simulink model "DisplayCANMsg"  (R2015a)
settings: Solver=ode45  StartTime=0.0  StopTime=10000000.0  RelTol=1e-3
settings Model: Creator=t430  LastModifiedBy=t430

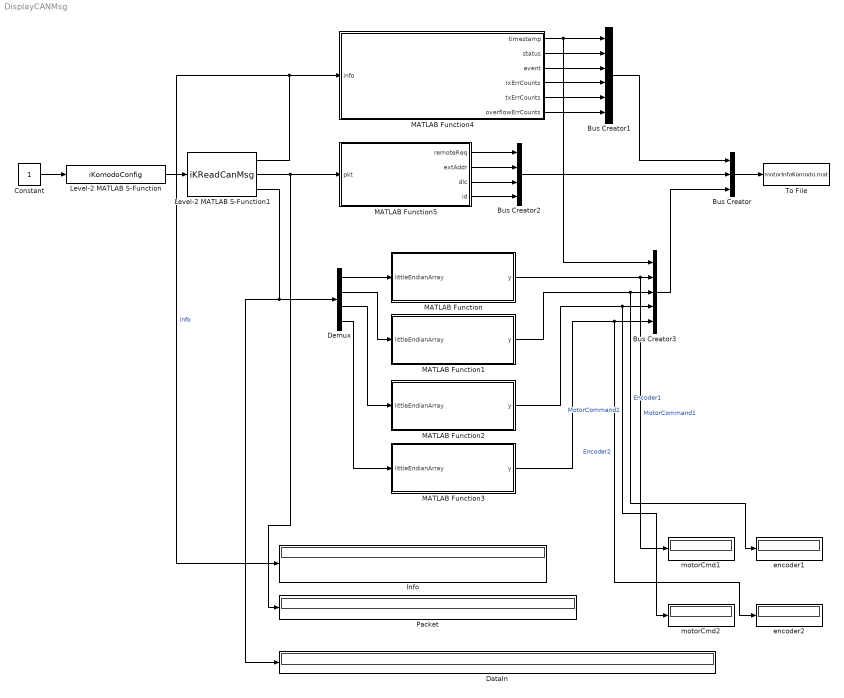
== system DisplayCANMsg ==
  Bus Creator : BusCreator  Inputs=3
  Bus Creator1 : BusCreator  Inputs=6
  Bus Creator2 : BusCreator
  Bus Creator3 : BusCreator  Inputs=5
  Constant : Constant  OutDataTypeStr=int32  SampleTime=0.001
  DataIn : Display
  Demux : Demux
  Info : Display
  Level-2 MATLAB S-Function : M-S-Function  FunctionName=iKomodoConfig  Parameters=0,1000000
  Level-2 MATLAB S-Function1 : M-S-Function  FunctionName=iKReadCanMsg
  MATLAB Function : MATLAB Function  TreatAsAtomicUnit=on
  MATLAB Function1 : MATLAB Function  TreatAsAtomicUnit=on
  MATLAB Function2 : MATLAB Function  TreatAsAtomicUnit=on
  MATLAB Function3 : MATLAB Function  TreatAsAtomicUnit=on
  MATLAB Function4 : MATLAB Function  TreatAsAtomicUnit=on
  MATLAB Function5 : MATLAB Function  TreatAsAtomicUnit=on
  Packet : Display
  To File : ToFile  Filename=motorInfoKomodo.mat  MatrixName=motorInfo  SaveFormat=Timeseries
  encoder1 : Display
  encoder2 : Display
  motorCmd1 : Display
  motorCmd2 : Display
  wires:
  Level-2 MATLAB S-Function/1 -> Level-2 MATLAB S-Function1/1
  Level-2 MATLAB S-Function1/1 -> Info/1, MATLAB Function4/1(info)  "info"
  Level-2 MATLAB S-Function1/2 -> MATLAB Function5/1(pkt), Packet/1
  Level-2 MATLAB S-Function1/3 -> Demux/1, DataIn/1
  Demux/1 -> MATLAB Function/1(littleEndianArray)
  MATLAB Function/1(y) -> motorCmd1/1, Bus Creator3/2  "MotorCommand1"
  Demux/2 -> MATLAB Function1/1(littleEndianArray)
  Demux/3 -> MATLAB Function2/1(littleEndianArray)
  Demux/4 -> MATLAB Function3/1(littleEndianArray)
  Constant/1 -> Level-2 MATLAB S-Function/1
  MATLAB Function1/1(y) -> encoder1/1, Bus Creator3/3  "Encoder1"
  MATLAB Function2/1(y) -> Bus Creator3/4, motorCmd2/1  "MotorCommand2"
  MATLAB Function3/1(y) -> Bus Creator3/5, encoder2/1  "Encoder2"
  Bus Creator/1 -> To File/1
  MATLAB Function4/6(overflowErrCounts) -> Bus Creator1/6
  MATLAB Function4/2(status) -> Bus Creator1/2
  MATLAB Function4/3(event) -> Bus Creator1/3
  MATLAB Function4/4(rxErrCounts) -> Bus Creator1/4
  MATLAB Function4/5(txErrCounts) -> Bus Creator1/5
  MATLAB Function5/1(remoteReq) -> Bus Creator2/1
  MATLAB Function5/2(extAddr) -> Bus Creator2/2
  MATLAB Function5/3(dlc) -> Bus Creator2/3
  MATLAB Function5/4(id) -> Bus Creator2/4
  Bus Creator1/1 -> Bus Creator/1
  Bus Creator2/1 -> Bus Creator/2
  MATLAB Function4/1(timestamp) -> Bus Creator1/1, Bus Creator3/1
  Bus Creator3/1 -> Bus Creator/3

== matlab function DisplayCANMsg/MATLAB Function1 ==
  data: littleEndianArray input; y output size=1
function y = ConvertBytesToInt16(littleEndianArray)
    y = typecast(uint8(littleEndianArray), 'int16');

== matlab function DisplayCANMsg/MATLAB Function ==
  data: littleEndianArray input; y output size=1
function y = ConvertBytesToInt16(littleEndianArray)
    y = typecast(uint8(littleEndianArray), 'int16');

== matlab function DisplayCANMsg/MATLAB Function2 ==
  data: littleEndianArray input; y output size=1
function y = ConvertBytesToInt16(littleEndianArray)
    y = typecast(uint8(littleEndianArray), 'int16');

== matlab function DisplayCANMsg/MATLAB Function3 ==
  data: littleEndianArray input; y output size=1
function y = ConvertBytesToInt16(littleEndianArray)
    y = typecast(uint8(littleEndianArray), 'int16');

== matlab function DisplayCANMsg/MATLAB Function4 ==
  data: info input; timestamp output; status output; event output; rxErrCounts output; txErrCounts output; overflowErrCounts output
function [timestamp,status,event,rxErrCounts, txErrCounts, overflowErrCounts] = komodoInfoStrExtractor(info)
    timestamp = double(info(1));
    status = info(2);
    event = info(3);
    rxErrCounts = info(7);
    txErrCounts = info(8);
    overflowErrCounts = info(9);

== matlab function DisplayCANMsg/MATLAB Function5 ==
  data: pkt input; remoteReq output; extAddr output; dlc output; id output
function [remoteReq,extAddr,dlc,id] = KomodoPacketStrExtractor(pkt)
    remoteReq = pkt(1);
    extAddr = pkt(2);
    dlc = pkt(3);
    id = pkt(4);
